simulink subsystem "GP2Y0A41"  (R2022b)
settings: Solver=VariableStepAuto  StartTime=0.0  StopTime=10.0  RelTol=1e-3
model mask{Pin=A0}
  mask prompts: Pin "svd:svd:PinPrompt"
libraries: mbedblockslib x1, dspstat3 x1
settings Model: Creator=micha  LastModifiedBy=micha

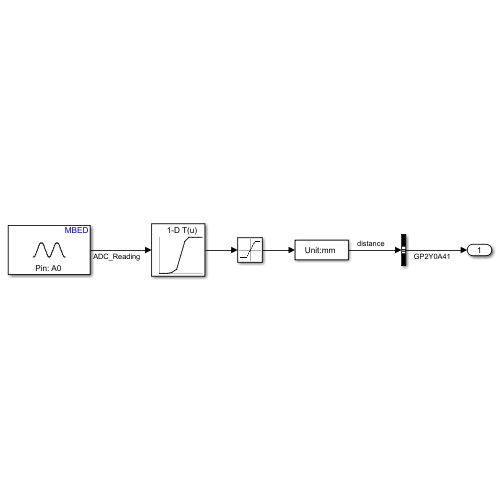
[thumbnail: Simulink's stored preview of the top-level diagram]
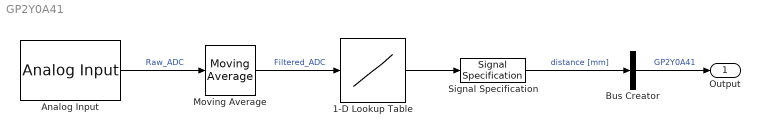
== system GP2Y0A41 ==
  1-D Lookup Table : Lookup_n-D  NumberOfTableDimensions=1  BreakpointsForDimension1=[0.0170, 0.0250, 0.0360, 0.0560, 0.0790, 0.1070, 0.1250, 0.1550, 0.2010, 0.2780, 0.3330, 0.4370, 0.6420, 0.8780]  Table=[600, 550, 500, 450, 400, 350, 300, 250, 200, 150, 125, 100, 70, 50]  InternalRulePriority=Speed  RndMeth=Simplest
  Analog Input : mbedblockslib/Analog Input  Pin=A1  ReadResultsOnly=off  ConversionTriggerSource=Software  ExternalTriggerType=uint32( 0 )  OutputDataType=double  EnableConversionCompleteNotify=off  EnableOuputStatus=off  SampleTime=-1
      settings: LibrarySourceBlock=stmnucleorootlib/Common/Analog Input
  Bus Creator : BusCreator  Inputs=1
  Moving Average : dspstat3/Moving Average  Method=Sliding window  ForgettingFactorPort=off  SpecifyWindowLength=on  WindowLength=20  OverlapLength=19  AllowArbitraryInputLength=off  ForgettingFactor=0.9  SimulateUsing=Code generation
  Signal Specification : SignalSpecification  Unit=mm
  Output : Outport
  wires:
  Bus Creator/1 -> Output/1  "GP2Y0A41"
  Moving Average/1 -> 1-D Lookup Table/1  "Filtered_ADC"
  Analog Input/1 -> Moving Average/1  "Raw_ADC"
  Signal Specification/1 -> Bus Creator/1  "distance [mm]"
  1-D Lookup Table/1 -> Signal Specification/1
